simulink model "Simulink_Practica_5"  (R2024b)
settings: Solver=VariableStepAuto  StartTime=0.0  StopTime=0.001  MaxStep=0.000001  RelTol=1e-3
settings Model: Creator=JUAN CARLOS

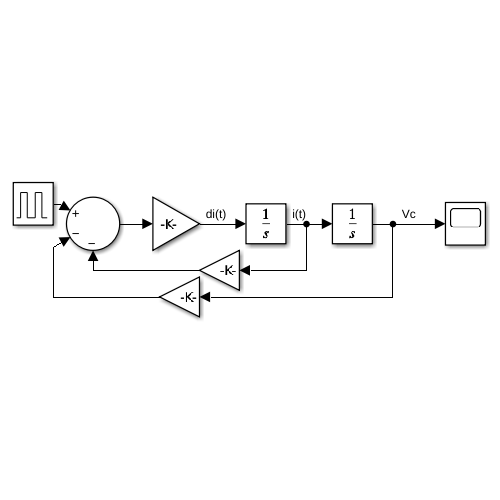
[thumbnail: Simulink's stored preview of the top-level diagram]
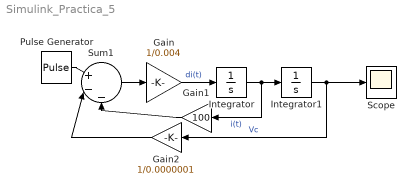
== system Simulink_Practica_5 ==
  Gain : Gain  Gain=1/0.004
  Gain1 : Gain  Gain=100
  Gain2 : Gain  Gain=1/0.0000001
  Integrator : Integrator
  Integrator1 : Integrator
  Pulse Generator : DiscretePulseGenerator  PulseType=Time based  Amplitude=9  Period=0.0022  PulseWidth=50
  Scope : Scope
  Sum1 : Sum  Inputs=|+--
  wires:
  Integrator/1 -> Gain1/1, Integrator1/1  "i(t)"
  Integrator1/1 -> Gain2/1, Scope/1  "Vc"
  Gain/1 -> Integrator/1  "di(t)"
  Sum1/1 -> Gain/1
  Pulse Generator/1 -> Sum1/1
  Gain1/1 -> Sum1/3
  Gain2/1 -> Sum1/2
